simulink model "prob3"  (R2020a)
settings: Solver=VariableStepAuto  StartTime=0.0  StopTime=10  MaxStep=0.001  RelTol=1e-3
values from neighbouring files (symbols this model uses):
  Noise = 628.31853071795865    [data.sldd]    (also in para.m = 628.318530718)
  OrigSign = 6283.1853071795858    [data.sldd]    (also in para.m = 6283.18530718)
settings Model: Creator=vijay  LastModifiedBy=vijay

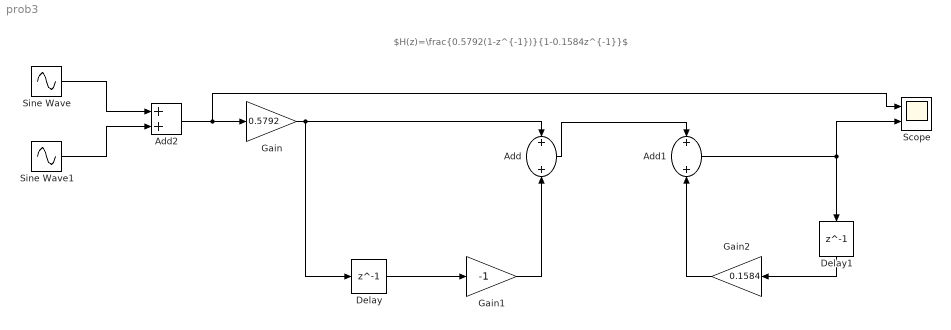
== system prob3 ==
  note: $H(z)=\frac{0.5792(1-z^{-1})}{1-0.1584z^{-1}}$
  Add : Sum
  Add1 : Sum
  Add2 : Sum
  Delay : Delay  DelayLength=1
  Delay1 : Delay  DelayLength=1
  Gain : Gain  Gain=0.5792
  Gain1 : Gain  Gain=-1
  Gain2 : Gain  Gain=0.1584
  Scope : Scope  NumInputPorts=2
  Sine Wave : Sin  Frequency=Noise  SampleTime=0
  Sine Wave1 : Sin  Frequency=OrigSign  SampleTime=0
  wires:
  Add2/1 -> Scope/1, Gain/1
  Gain/1 -> Delay/1, Add/1
  Delay/1 -> Gain1/1
  Gain1/1 -> Add/2
  Add/1 -> Add1/1
  Add1/1 -> Delay1/1, Scope/2
  Delay1/1 -> Gain2/1
  Gain2/1 -> Add1/2
  Sine Wave/1 -> Add2/1
  Sine Wave1/1 -> Add2/2
